simulink model "w1prob2"  (R2020a)
settings: Solver=VariableStepAuto  StartTime=0.0  StopTime=10.0  RelTol=1e-3
PostLoadFcn:
  | M1 = 2500;
  | M2 = 320;
  | K1 = 80000;
  | K2 = 500000;
  | b = 350;
settings Model: Creator=Anjali123  LastModifiedBy=Anjali123

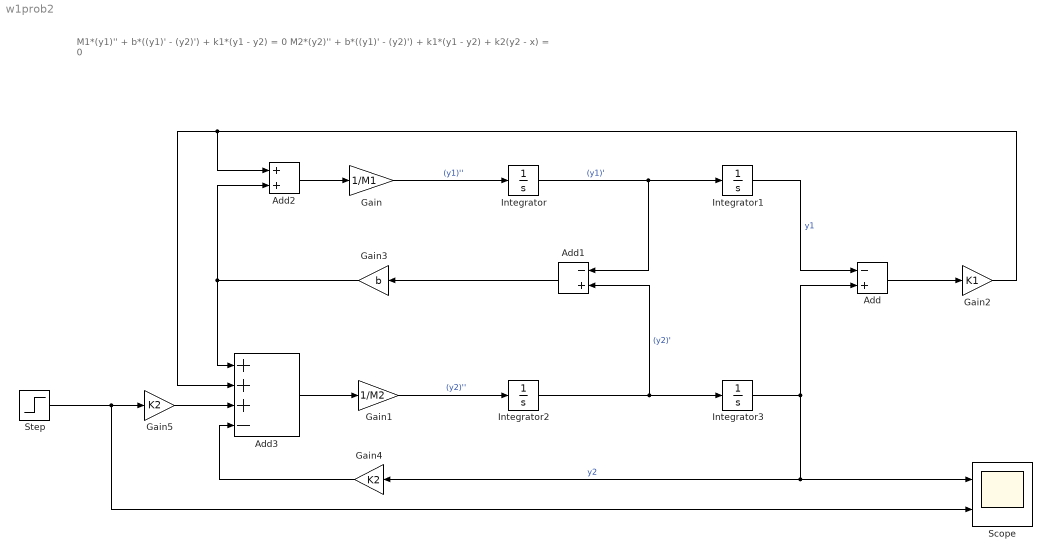
== system w1prob2 ==
  note: M1*(y1)'' + b*((y1)' - (y2)') + k1*(y1 - y2) = 0
      | M2*(y2)'' + b*((y1)' - (y2)') + k1*(y1 - y2) + k2(y2 - x) = 0
  Add : Sum  Inputs=-+
  Add1 : Sum  Inputs=-+
  Add2 : Sum
  Add3 : Sum  Inputs=+++-
  Gain : Gain  Gain=1/M1
  Gain1 : Gain  Gain=1/M2
  Gain2 : Gain  Gain=K1
  Gain3 : Gain  Gain=b
  Gain4 : Gain  Gain=K2
  Gain5 : Gain  Gain=K2
  Integrator{,1..3} (4 alike) : Integrator
  Scope : Scope  NumInputPorts=2
  Step : Step  SampleTime=0
  wires:
  Gain/1 -> Integrator/1  "(y1)''"
  Integrator/1 -> Add1/1, Integrator1/1  "(y1)'"
  Integrator1/1 -> Add/1  "y1"
  Gain1/1 -> Integrator2/1  "(y2)''"
  Integrator2/1 -> Add1/2, Integrator3/1  "(y2)'"
  Integrator3/1 -> Add/2, Gain4/1, Scope/1  "y2"
  Add/1 -> Gain2/1
  Add1/1 -> Gain3/1
  Add2/1 -> Gain/1
  Gain3/1 -> Add3/1, Add2/2
  Gain2/1 -> Add3/2, Add2/1
  Add3/1 -> Gain1/1
  Gain4/1 -> Add3/4
  Step/1 -> Scope/2, Gain5/1
  Gain5/1 -> Add3/3
